simulink model "PlantaPadrao"  (R2019a)
settings: Solver=VariableStepAuto  StartTime=0.0  StopTime=10  RelTol=1e-3
undefined symbols (not defined in the file): A, B, C
settings Model: Creator=Cliente  LastModifiedBy=Cliente

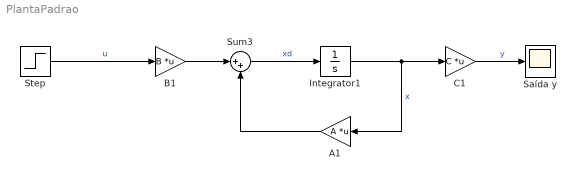
== system PlantaPadrao ==
  A1 : Gain  Gain=A  Multiplication=Matrix(K*u) (u vector)
  B1 : Gain  Gain=B  Multiplication=Matrix(K*u)
  C1 : Gain  Gain=C  Multiplication=Matrix(K*u) (u vector)
  Integrator1 : Integrator
  Saída y : Scope
  Step : Step  SampleTime=0
  Sum3 : Sum  Inputs=|++
  wires:
  Integrator1/1 -> A1/1, C1/1  "x"
  Sum3/1 -> Integrator1/1  "xd"
  A1/1 -> Sum3/2
  Step/1 -> B1/1  "u"
  B1/1 -> Sum3/1
  C1/1 -> Saída y/1  "y"
